simulink subsystem "TechnicMotor"  (R2023b)
settings: Solver=VariableStepAuto  StartTime=0.0  StopTime=10.0  RelTol=1e-3
undefined symbols (not defined in the file): J
libraries: fl_lib x6, ee_lib x3, nesl_utility x3
settings Model: Creator=zuhai  LastModifiedBy=zuhai

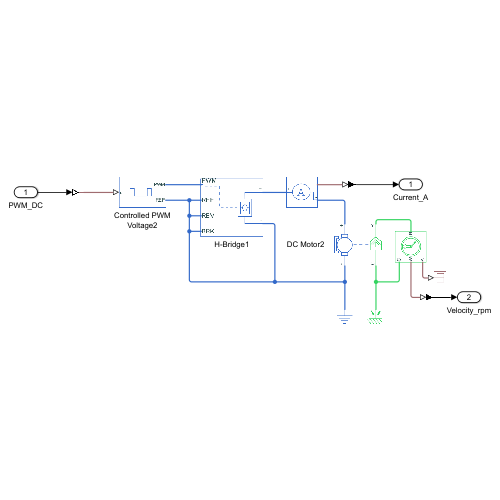
[thumbnail: Simulink's stored preview of the top-level diagram]
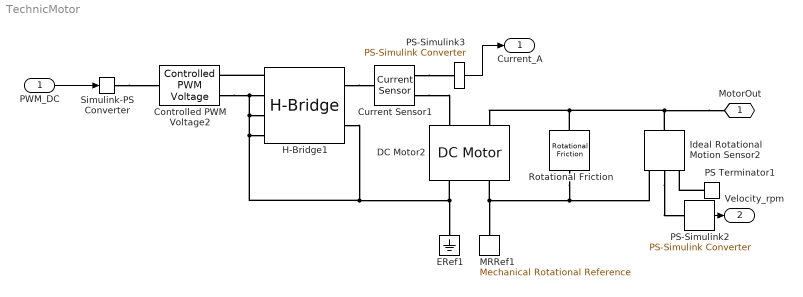
== system TechnicMotor ==
  PWM_DC : Inport
  Controlled PWM Voltage2 : ee_lib/Integrated Circuits/Controlled PWM Voltage  F=4000 Hz  TD=0 s  pulse_width_offset=0 s  pulse_min=0 s  pwm_or_av=ee.enum.pwm_or_av.averaged  event_type=1  sample_time=5e-6 s  Vmin=0 V  Vmax=5 V  Vm=5 V  u_min=0  u_max=1
      settings: InternalSimscapePortConfiguration="{\"Bottom\":[],\"Left\":[{\"id\":\"u\",\"label\":\"u\",\"type\":\"input\"}],\"Right\":[{\"id\":\"p2\",\"label\":\"PWM\",\"type\":\"foundation.electrical.electrical\"},{\"id\":\"n2\",\"label\":\"REF\",\"type\":\"foundation.electrical.electrical\"}],\"Top\":[]}"
  Current Sensor1 : fl_lib/Electrical/Electrical Sensors/Current Sensor
  DC Motor2 : ee_lib/Electromechanical/Brushed Motors/DC Motor  field_option=ee.enum.field_option.pm  Rf=100 Ohm  Lf=1 H  Laf=0.15 H  If0=0 A  parameterization=ee.enum.dcparam_option.circuit_param  Ra=resistance_mean_ohm Ohm  La=L H  emf_or_torque=1  Kv=r_m V/(rad/s)  Ki=6.876e-04 N*m/A  T_stall=0.1 N*m  w_max=4000 rpm  w_rated=2500 rpm  P_rated=10 W  V_rated=12 V  lam_param=1  i_noload=0 A  V_i_noload=1.5 V  J=J kg*m^2  lam=0 N*m/(rad/s)  speed0=0 rpm  enable_fault_armature=simscape.enum.onoff.off  rev_faulted=1 / 3  G_faulted_armature=1e-5 S  fault_trigger_armature=ee.enum.faults.faultTrigger.temporal  t_fault_armature=1 s  max_permissible_current_armature=inf A  t_fail_on_current_armature=1 s  enable_fault_field=simscape.enum.onoff.off  G_faulted_field=1e-5 S  fault_trigger_field=ee.enum.faults.faultTrigger.temporal  t_fault_field=1 s  max_permissible_current_field=inf A  t_fail_on_current_field=1 s  fault_action=simscape.enum.assert.action.none  alpha=3.93e-3 1/K  Tmeas=25 degC  thermal_mass=100 J/K  initial_temperature=25 degC
  ERef1 : fl_lib/Electrical/Electrical Elements/Electrical Reference
  H-Bridge1 : ee_lib/Semiconductors & Converters/Converters/H-Bridge  supply_ports=ee.enum.supply_ports.hidesupply  pwm_or_av=2  regenerative_braking_mode=ee.enum.converters.regenerative_braking_mode.always_enabled  discontinuous=0  freewheeling_mode=1  Rload=3.38+0.1 Ohm  Lload=1e-5 H  F=4 kHz  Venable=2.5 V  Vmax=5 V  Vreverse=2.5 V  Vbrake=2.5 V  Vm=battery_voltage_V V  Ron=0.1 Ohm  Don=0.1 Ohm  Goff=1e-6 S  Tmeas=298.15 K  Ron2=0.1 Ohm  Don2=0.05 Ohm  Tmeas2=398.15 K  thermal_mass=100 J/K  initial_temperature=298.15 K
  Ideal Rotational Motion Sensor2 : fl_lib/Mechanical/Mechanical Sensors/Ideal Rotational Motion Sensor  reference=foundation.enum.MeasurementReference.difference  acceleration_port=false  velocity_port=true  position_port=true  wrap_angle=simscape.enum.onoff.off  offset=0 deg
  MRRef1 : fl_lib/Mechanical/Rotational Elements/Mechanical Rotational Reference
  PS Terminator1 : fl_lib/Physical Signals/Sinks/PS Terminator
  PS-Simulink2 : nesl_utility/PS-Simulink Converter  PhysicalDomain=network_engine_domain  SubClassName=ps_output  LeftPortType=input  RightPortType=output  PseudoPeriodic=off  Frequencies=[]  VectorFormat=1-D array  Unit=rpm  AffineConversion=off
  PS-Simulink3 : nesl_utility/PS-Simulink Converter  PhysicalDomain=network_engine_domain  SubClassName=ps_output  LeftPortType=input  RightPortType=output  PseudoPeriodic=off  Frequencies=[]  VectorFormat=1-D array  Unit=A  AffineConversion=off
  Rotational Friction : fl_lib/Mechanical/Rotational Elements/Rotational Friction  brkwy_trq=breakaway_torque N*m  brkwy_vel=0.1 rad/s  Col_trq=breakaway_torque N*m  visc_coef=B_m N*m*s/rad  w_specify=off  w_priority=None  w=0 rad/s  w_nominal_specify=off  w_nominal_unit=rad/s  w_nominal_value=1  t_specify=off  t_priority=None  t=0 N*m  t_nominal_specify=off  t_nominal_unit=N*m  t_nominal_value=1
  Simulink-PS Converter : nesl_utility/Simulink-PS Converter  PhysicalDomain=network_engine_domain  SubClassName=ps_input  LeftPortType=input  RightPortType=output  PseudoPeriodic=off  Frequencies=[]  NoiseDistribution=none  NoiseParameters=[]  Unit=1  AffineConversion=off  FilteringAndDerivatives=provide  SimscapeFilterOrder=1  InputFilterTimeConstant=0.001  UdotUserProvided=0
  MotorOut : PMIOPort  Side=Left
  Current_A : Outport
  Velocity_rpm : Outport  Port=2
  wires:
  PS-Simulink3/1 -> Current_A/1
  PS-Simulink2/1 -> Velocity_rpm/1
  PWM_DC/1 -> Simulink-PS Converter/1
  connections:
  Rotational Friction/LConn1 -- MRRef1/LConn1 -- DC Motor2/RConn2 -- Ideal Rotational Motion Sensor2/RConn1
  Controlled PWM Voltage2/RConn2 -- DC Motor2/RConn1 -- ERef1/LConn1 -- H-Bridge1/RConn2 -- H-Bridge1/LConn4 -- H-Bridge1/LConn3 -- H-Bridge1/LConn2
  MotorOut/RConn1 -- Rotational Friction/RConn1 -- DC Motor2/LConn2 -- Ideal Rotational Motion Sensor2/LConn1
  H-Bridge1/LConn1 -- Controlled PWM Voltage2/RConn1
  Current Sensor1/RConn1 -- PS-Simulink3/LConn1
  Current Sensor1/RConn2 -- DC Motor2/LConn1
  PS Terminator1/LConn1 -- Ideal Rotational Motion Sensor2/RConn3
  Ideal Rotational Motion Sensor2/RConn2 -- PS-Simulink2/LConn1
  H-Bridge1/RConn1 -- Current Sensor1/LConn1
  Simulink-PS Converter/RConn1 -- Controlled PWM Voltage2/LConn1
